simulink subsystem "steeringWheel"  (R2023b)
settings: Solver=VariableStepAuto  StartTime=0.0  StopTime=10.0  RelTol=1e-3
libraries: steeringWheel_lib x5, Raptor_lib x5
settings Model: Creator=serga  LastModifiedBy=serga
settings OptimizationCC: ReuseModelBlockBuffer=off

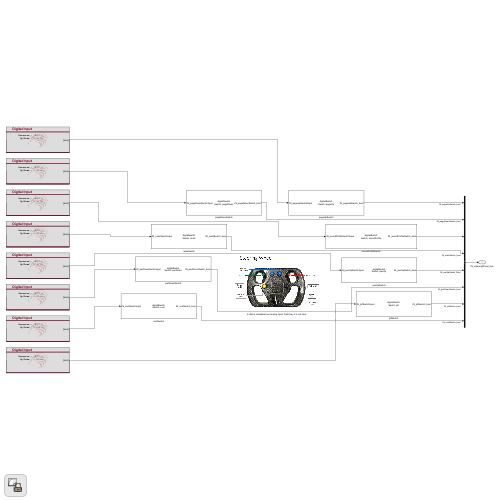
[thumbnail: Simulink's stored preview of the top-level diagram]
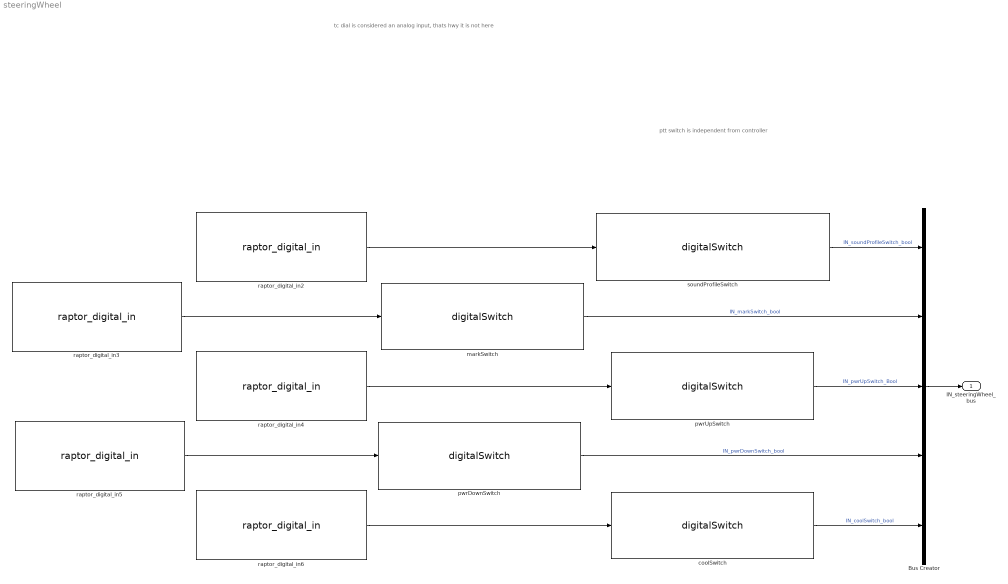
== system steeringWheel ==
  note: ptt switch is independent from controller
  note: tc dial is considered an analog input, thats hwy it is not here
  Bus Creator : BusCreator  Inputs=5
  coolSwitch : steeringWheel_lib/digitalSwitch  pos='cool'
  markSwitch : steeringWheel_lib/digitalSwitch  pos='mark'
  pwrDownSwitch : steeringWheel_lib/digitalSwitch  pos='pwrDown'
  pwrUpSwitch : steeringWheel_lib/digitalSwitch  pos='pwrUp'
  raptor_digital_in2 : Raptor_lib/Input & Output/raptor_digital_in  resourceValues=WAKE_INPUT1|INPUT33|INPUT34|INPUT35|INPUT36|INPUT37|INPUT38|INPUT39|INPUT40|(None)  resource=INPUT35  pullUDValues=1.3k PD  pullUD=1.3k PD  upperThres='RAPTOR MASK DEFAULT'  lowerThres='RAPTOR MASK DEFAULT'
      settings: SourceProductName=Raptor
  raptor_digital_in3 : Raptor_lib/Input & Output/raptor_digital_in  resourceValues=WAKE_INPUT1|INPUT33|INPUT34|INPUT35|INPUT36|INPUT37|INPUT38|INPUT39|INPUT40|(None)  resource=INPUT37  pullUDValues=1.3k PU  pullUD=1.3k PU  upperThres='RAPTOR MASK DEFAULT'  lowerThres='RAPTOR MASK DEFAULT'
      settings: SourceProductName=Raptor
  raptor_digital_in4 : Raptor_lib/Input & Output/raptor_digital_in  resourceValues=WAKE_INPUT1|INPUT33|INPUT34|INPUT35|INPUT36|INPUT37|INPUT38|INPUT39|INPUT40|(None)  resource=INPUT40  pullUDValues=1.3k PU  pullUD=1.3k PU  upperThres='RAPTOR MASK DEFAULT'  lowerThres='RAPTOR MASK DEFAULT'
      settings: SourceProductName=Raptor
  raptor_digital_in5 : Raptor_lib/Input & Output/raptor_digital_in  resourceValues=WAKE_INPUT1|INPUT33|INPUT34|INPUT35|INPUT36|INPUT37|INPUT38|INPUT39|INPUT40|(None)  resource=INPUT39  pullUDValues=1.3k PU  pullUD=1.3k PU  upperThres='RAPTOR MASK DEFAULT'  lowerThres='RAPTOR MASK DEFAULT'
      settings: SourceProductName=Raptor
  raptor_digital_in6 : Raptor_lib/Input & Output/raptor_digital_in  resourceValues=WAKE_INPUT1|INPUT33|INPUT34|INPUT35|INPUT36|INPUT37|INPUT38|INPUT39|INPUT40|(None)  resource=INPUT38  pullUDValues=1.18k PU  pullUD=1.18k PU  upperThres='RAPTOR MASK DEFAULT'  lowerThres='RAPTOR MASK DEFAULT'
      settings: SourceProductName=Raptor
  soundProfileSwitch : steeringWheel_lib/digitalSwitch  pos='soundProfile'
  IN_steeringWheel_bus : Outport
  wires:
  Bus Creator/1 -> IN_steeringWheel_bus/1
  coolSwitch/1 -> Bus Creator/5  "IN_coolSwitch_bool"
  pwrDownSwitch/1 -> Bus Creator/4  "IN_pwrDownSwitch_bool"
  markSwitch/1 -> Bus Creator/2  "IN_markSwitch_bool"
  soundProfileSwitch/1 -> Bus Creator/1  "IN_soundProfileSwitch_bool"
  pwrUpSwitch/1 -> Bus Creator/3  "IN_pwrUpSwitch_Bool"
  raptor_digital_in2/1 -> soundProfileSwitch/1
  raptor_digital_in3/1 -> markSwitch/1
  raptor_digital_in4/1 -> pwrUpSwitch/1
  raptor_digital_in5/1 -> pwrDownSwitch/1
  raptor_digital_in6/1 -> coolSwitch/1
